simulink model "test_mechanics"  (R2017a)
settings: Solver=VariableStepAuto  StartTime=0.0  StopTime=2*pi()  MaxStep=1e-3  RelTol=1e-3
libraries: slidercrank_basic_library_v1 x7, simulink x1
settings Model: Creator=filip  LastModifiedBy=filip

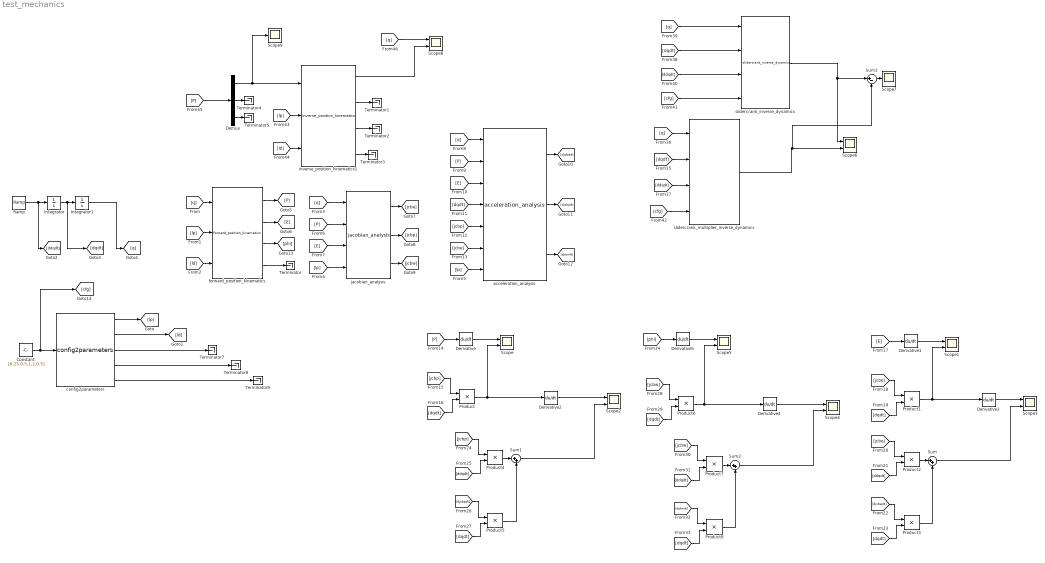
== system test_mechanics ==
  Constant : Constant  Value=[0.25,0.5,1,2,0.5]
  Demux : Demux  Outputs=3
  Derivative{,1..5} (6 alike) : Derivative
  Integrator : Integrator
  Integrator1 : Integrator
  Product{,1..8} (9 alike) : Product
  Ramp : simulink/Sources/Ramp  slope=1  start=0  X0=0
  Scope{,1..6,8} (8 alike) : Scope  NumInputPorts=2
  Scope7 : Scope
  Scope9 : Scope
  Sum : Sum  Inputs=|++
  Sum1 : Sum  Inputs=|++
  Sum2 : Sum  Inputs=|++
  Sum3 : Sum  Inputs=|+-
  Terminator{,1..5,7..9} (9 alike) : Terminator
  acceleration_analysis : slidercrank_basic_library_v1/acceleration_analysis
  config2parameters : slidercrank_basic_library_v1/config2parameters
  forward_position_kinematics : slidercrank_basic_library_v1/forward_position_kinematics
  inverse_position_kinematics1 : slidercrank_basic_library_v1/inverse_position_kinematics
  jacobian_analysis : slidercrank_basic_library_v1/jacobian_analysis
  slidercrank_inverse_dynamics : slidercrank_basic_library_v1/slidercrank_inverse_dynamics
  slidercrank_multiplier_inverse_dynamics : slidercrank_basic_library_v1/slidercrank_multiplier_inverse_dynamics
  wires:
  Constant/1 -> [cfg], config2parameters/1
  config2parameters/3 -> Terminator7/1
  config2parameters/4 -> Terminator8/1
  config2parameters/5 -> Terminator9/1
  config2parameters/1 -> [lp]
  config2parameters/2 -> [ld]
  Ramp/1 -> [ddqdt], Integrator/1
  Integrator/1 -> [dqdt], Integrator1/1
  Integrator1/1 -> [q]
  [q] -> forward_position_kinematics/1
  [lp] -> forward_position_kinematics/2
  [ld] -> forward_position_kinematics/3
  [q] -> jacobian_analysis/1
  [lp] -> jacobian_analysis/4
  [lp] -> acceleration_analysis/7
  forward_position_kinematics/1 -> [P]
  forward_position_kinematics/2 -> [E]
  [P] -> jacobian_analysis/2
  [E] -> jacobian_analysis/3
  [q] -> acceleration_analysis/1
  [P] -> acceleration_analysis/2
  [E] -> acceleration_analysis/3
  jacobian_analysis/1 -> [jcbe]
  jacobian_analysis/2 -> [jcbp]
  jacobian_analysis/3 -> [jcbw]
  [dqdt] -> acceleration_analysis/4
  [jcbp] -> acceleration_analysis/5
  [jcbe] -> acceleration_analysis/6
  acceleration_analysis/3 -> [djcbwdt]
  acceleration_analysis/1 -> [djcbedt]
  acceleration_analysis/2 -> [djcbpdt]
  [P] -> Derivative/1
  Derivative/1 -> Scope/1
  Product/1 -> Derivative2/1, Scope/2
  [jcbp] -> Product/1
  [dqdt] -> Product/2
  Product1/1 -> Derivative3/1, Scope1/2
  [E] -> Derivative1/1
  [dqdt] -> Product1/2
  [jcbe] -> Product1/1
  Derivative1/1 -> Scope1/1
  Derivative2/1 -> Scope2/1
  Derivative3/1 -> Scope3/1
  [ddqdt] -> Product2/2
  [jcbe] -> Product2/1
  [djcbedt] -> Product3/1
  [dqdt] -> Product3/2
  Product2/1 -> Sum/1
  Product3/1 -> Sum/2
  Sum/1 -> Scope3/2
  [djcbpdt] -> Product5/1
  Product5/1 -> Sum1/2
  Sum1/1 -> Scope2/2
  [dqdt] -> Product5/2
  Product4/1 -> Sum1/1
  [jcbp] -> Product4/1
  [ddqdt] -> Product4/2
  [jcbw] -> Product6/1
  [dqdt] -> Product6/2
  Sum2/1 -> Scope4/2
  [jcbw] -> Product7/1
  [ddqdt] -> Product7/2
  Product8/1 -> Sum2/2
  [dqdt] -> Product8/2
  [djcbwdt] -> Product8/1
  Product7/1 -> Sum2/1
  Derivative4/1 -> Scope4/1
  [phi] -> Derivative5/1
  Derivative5/1 -> Scope5/1
  Product6/1 -> Scope5/2, Derivative4/1
  forward_position_kinematics/4 -> Terminator/1
  forward_position_kinematics/3 -> [phi]
  [q] -> slidercrank_multiplier_inverse_dynamics/1
  [dqdt] -> slidercrank_multiplier_inverse_dynamics/2
  [cfg] -> slidercrank_multiplier_inverse_dynamics/4
  [ddqdt] -> slidercrank_multiplier_inverse_dynamics/3
  [q] -> slidercrank_inverse_dynamics/1
  [dqdt] -> slidercrank_inverse_dynamics/2
  [ddqdt] -> slidercrank_inverse_dynamics/3
  [cfg] -> slidercrank_inverse_dynamics/4
  slidercrank_inverse_dynamics/1 -> Sum3/1, Scope6/1
  slidercrank_multiplier_inverse_dynamics/1 -> Sum3/2, Scope6/2
  Sum3/1 -> Scope7/1
  [lp] -> inverse_position_kinematics1/2
  [ld] -> inverse_position_kinematics1/3
  inverse_position_kinematics1/2 -> Terminator1/1
  inverse_position_kinematics1/3 -> Terminator2/1
  inverse_position_kinematics1/4 -> Terminator3/1
  [P] -> Demux/1
  Demux/1 -> Scope9/1, inverse_position_kinematics1/1
  Demux/2 -> Terminator4/1
  Demux/3 -> Terminator5/1
  inverse_position_kinematics1/1 -> Scope8/2
  [q] -> Scope8/1
